simulink model "Prob04"  (R2020a)
settings: Solver=ode15s  StartTime=0.0  StopTime=0.2  RelTol=1e-3
values from neighbouring files (symbols this model uses):
  b = 3.5077E-6    [Dictionary_data.sldd]
  J = 3.2284E-6    [Dictionary_data.sldd]
  K = 0.0274    [Dictionary_data.sldd]
  L = 2.75E-6    [Dictionary_data.sldd]
  R = 4.0    [Dictionary_data.sldd]
undefined symbols (not defined in the file or in its folder): Kd, Ki, Kp
settings Model: DataDictionary=Dictionary_data.sldd  Creator=Shivam  LastModifiedBy=Shivam

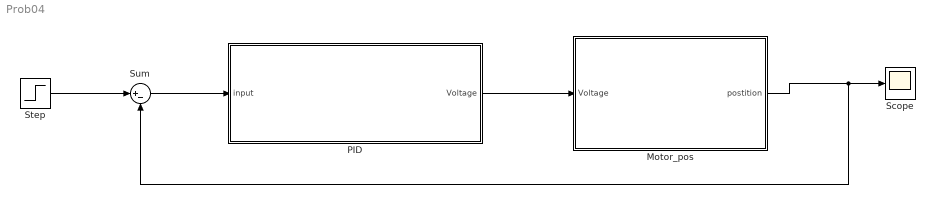
== system Prob04 ==
  Motor_pos : Subsystem
  PID : Subsystem
  Scope : Scope
  Step : Step  Time=0  SampleTime=0
  Sum : Sum  Inputs=|+-
  wires:
  Motor_pos/1(postition) -> Sum/2, Scope/1
  Sum/1 -> PID/1(input)
  PID/1(Voltage) -> Motor_pos/1(Voltage)
  Step/1 -> Sum/1

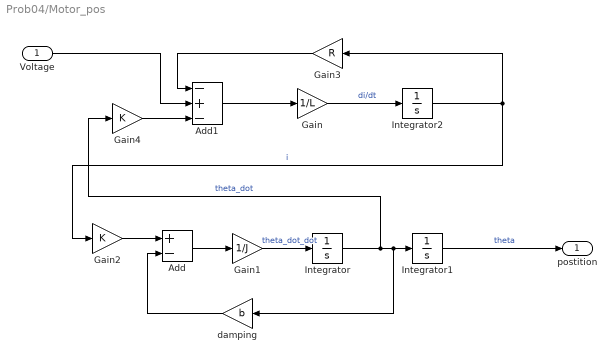
== system Prob04/Motor_pos ==
  Voltage : Inport
  Add : Sum  Inputs=+-
  Add1 : Sum  Inputs=-+-
  Gain : Gain  Gain=1/L
  Gain1 : Gain  Gain=1/J
  Gain2 : Gain  Gain=K
  Gain3 : Gain  Gain=R
  Gain4 : Gain  Gain=K
  Integrator : Integrator
  Integrator1 : Integrator
  Integrator2 : Integrator
  damping : Gain  Gain=b
  postition : Outport
  wires:
  Integrator1/1 -> postition/1  "theta"
  Integrator/1 -> Gain4/1, damping/1, Integrator1/1  "theta_dot"
  Voltage/1 -> Add1/2
  Gain2/1 -> Add/1
  Add1/1 -> Gain/1
  Gain1/1 -> Integrator/1  "theta_dot_dot"
  Integrator2/1 -> Gain3/1, Gain2/1  "i"
  Add/1 -> Gain1/1
  Gain/1 -> Integrator2/1  "di/dt"
  Gain3/1 -> Add1/1
  damping/1 -> Add/2
  Gain4/1 -> Add1/3

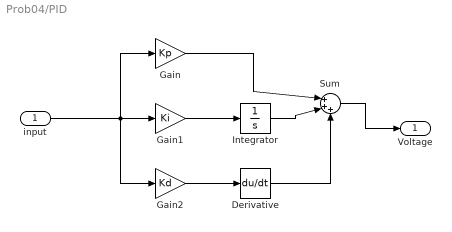
== system Prob04/PID ==
  input : Inport
  Derivative : Derivative
  Gain : Gain  Gain=Kp
  Gain1 : Gain  Gain=Ki
  Gain2 : Gain  Gain=Kd
  Integrator : Integrator
  Sum : Sum  Inputs=|+++
  Voltage : Outport
  wires:
  Gain1/1 -> Integrator/1
  Gain2/1 -> Derivative/1
  Gain/1 -> Sum/1
  Integrator/1 -> Sum/2
  Derivative/1 -> Sum/3
  input/1 -> Gain2/1, Gain1/1, Gain/1
  Sum/1 -> Voltage/1
